simulink model "pendule_inv_etu"  (R2017a)
settings: Solver=VariableStepAuto  StartTime=t0  StopTime=tf  RelTol=1e-3
undefined symbols (not defined in the file): g, K, l, ue, x0, xe
settings Model: Creator=cmaurice  LastModifiedBy=cmaurice

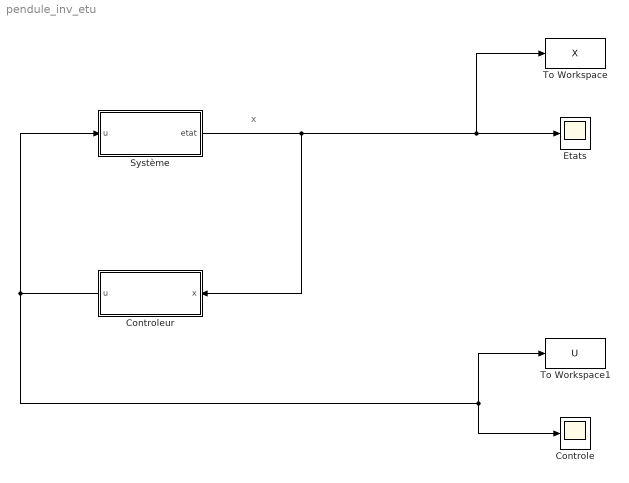
== system pendule_inv_etu ==
  note: x
  Controle : Scope
  Controleur : Subsystem
  Etats : Scope
  "Système " : Subsystem
  To Workspace : ToWorkspace  VariableName=X  SaveFormat=Timeseries  SampleTime=-1
  To Workspace1 : ToWorkspace  VariableName=U  SaveFormat=Timeseries  SampleTime=-1
  wires:
  Controleur/1(u) -> To Workspace1/1, Controle/1, "Système "/1(u)
  "Système "/1(etat) -> To Workspace/1, Etats/1, Controleur/1(x)

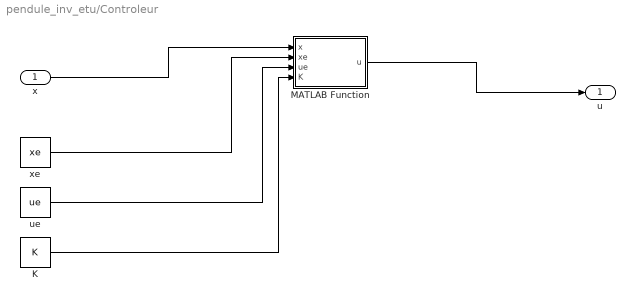
== system pendule_inv_etu/Controleur ==
  x : Inport
  K : Constant  Value=K
  MATLAB Function : MATLAB Function  TreatAsAtomicUnit=on
  ue : Constant  Value=ue
  xe : Constant  Value=xe
  u : Outport
  wires:
  x/1 -> MATLAB Function/1(x)
  MATLAB Function/1(u) -> u/1
  xe/1 -> MATLAB Function/2(xe)
  ue/1 -> MATLAB Function/3(ue)
  K/1 -> MATLAB Function/4(K)

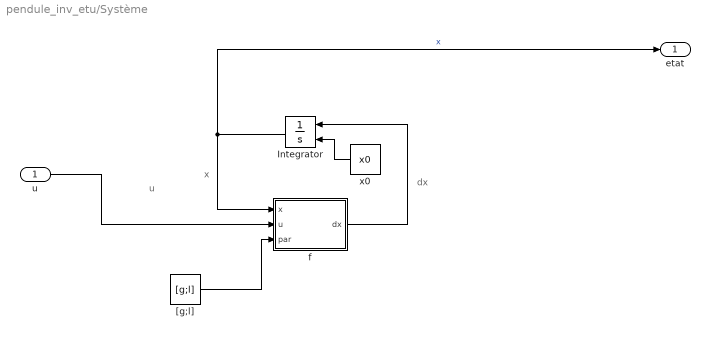
== system pendule_inv_etu/Système  ==
  note: u
  note: x
  note: dx
  u : Inport
  Integrator : Integrator  InitialConditionSource=external
  "[g;l] " : Constant  Value=[g;l]
  f : MATLAB Function  TreatAsAtomicUnit=on
  "x0 " : Constant  Value=x0
  etat : Outport
  wires:
  u/1 -> f/2(u)
  "[g;l] "/1 -> f/3(par)
  f/1(dx) -> Integrator/1
  Integrator/1 -> etat/1, f/1(x)  "x"
  "x0 "/1 -> Integrator/2

== matlab function pendule_inv_etu/Système /f ==
  data: x input; u input; dx output; par input
function dx = fcn(x,u,par)
g = par(1);
l = par(2);
dx = [x(2); (g/l)*sin(x(1))-(cos(x(1))*u)/l];

== matlab function pendule_inv_etu/Controleur/MATLAB Function ==
  data: x input; u output; xe input; ue input; K input
function u = fcn(x,xe,ue,K)
u = ue + K(:)'*(x(:)-xe(:));
